simulink library "INT_APP_Kickdown"  (R2016b)
settings: Solver=VariableStepAuto  StartTime=0.0  StopTime=10.0  RelTol=1e-3
settings Model: Creator=Administrator  LastModifiedBy=Administrator

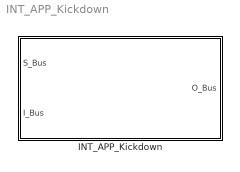
== system INT_APP_Kickdown ==
  INT_APP_Kickdown : Subsystem

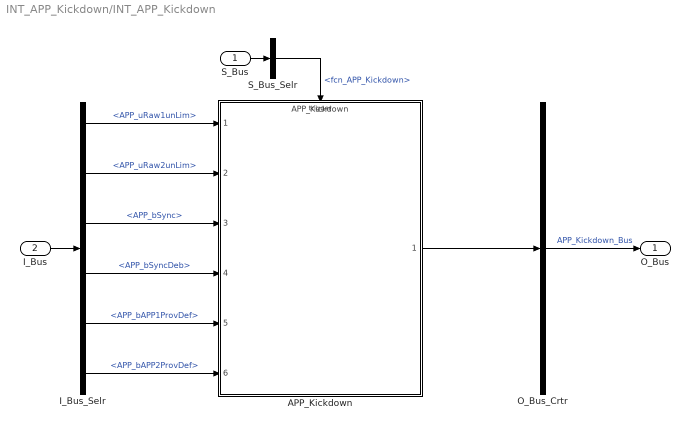
== system INT_APP_Kickdown/INT_APP_Kickdown ==
  S_Bus : Inport
  I_Bus : Inport  Port=2
  APP_Kickdown : ModelReference  ModelNameDialog=APP_Kickdown  SimulationMode=Normal  ModelReferenceVersion=1.8  TriggerPortName=function  TriggerPortTriggerType=function-call  TriggerPortStatesWhenEnabling=held
  I_Bus_Selr : BusSelector  OutputSignals=APP_uRaw1unLim,APP_uRaw2unLim,APP_bSync,APP_bSyncDeb,APP_bAPP1ProvDef,APP_bAPP2ProvDef
  O_Bus_Crtr : BusCreator  Inputs=1
  S_Bus_Selr : BusSelector  OutputSignals=fcn_APP_Kickdown
  O_Bus : Outport
  wires:
  S_Bus_Selr/1 -> APP_Kickdown/Trigger  "<fcn_APP_Kickdown>"
  S_Bus/1 -> S_Bus_Selr/1
  I_Bus/1 -> I_Bus_Selr/1
  I_Bus_Selr/1 -> APP_Kickdown/1  "<APP_uRaw1unLim>"
  I_Bus_Selr/2 -> APP_Kickdown/2  "<APP_uRaw2unLim>"
  I_Bus_Selr/3 -> APP_Kickdown/3  "<APP_bSync>"
  I_Bus_Selr/4 -> APP_Kickdown/4  "<APP_bSyncDeb>"
  I_Bus_Selr/5 -> APP_Kickdown/5  "<APP_bAPP1ProvDef>"
  I_Bus_Selr/6 -> APP_Kickdown/6  "<APP_bAPP2ProvDef>"
  O_Bus_Crtr/1 -> O_Bus/1  "APP_Kickdown_Bus"
  APP_Kickdown/1 -> O_Bus_Crtr/1
